simulink model "sim_dinamica"  (R2020a)
settings: Solver=VariableStepAuto  StartTime=0.0  StopTime=15  RelTol=1e-3
values from neighbouring files (symbols this model uses):
  theta_initial = [0 pi/2 -pi/2 0 0]    [teste_dinamica.m]
  torque_final = [0 0 0 0 0]    [teste_dinamica.m]
  torque_initial = [0 0 0 0 0]    [teste_dinamica.m]
  torque_step_time = [0 0 0 0 0]    [teste_dinamica.m]
(part 3 of 3)

== matlab function sim_dinamica/MATLAB Function ==
  data: dTh input; F output
function F = calcul_F(dTh)

F = 0.3*dTh;
